simulink model "ROPOD_Control_Control_SIM"  (R2017b)
settings: Solver=VariableStepAuto  StartTime=0.0  StopTime=inf  RelTol=1e-3
values from neighbouring files (symbols this model uses):
  FFtheta_intia = 0    [init_model.m]
  FFxy_mass = 0*80    (= 0)    [init_model.m]
  flock_FFtheta_friction = 50    [init_model.m]
  flock_FFxy_friction = 100    [init_model.m]
  I_fhz_ddelta_cntr = 0    [init_model.m]
  I_fhz_dtheta_cntr = 0.3    [init_model.m]
  I_fhz_dtheta_flock_cntr = 0.1    [init_model.m]
  I_fhz_dvarphi_cntr = 0    [init_model.m]
  I_fhz_dxdy_cntr = 0.25    [init_model.m]
  I_fhz_dxdy_flock_cntr = 0.1    [init_model.m]
  K_gain_ddelta_cntr = 0.1    [init_model.m]
  K_gain_dtheta_cntr = 150    [init_model.m]
  K_gain_dtheta_flock_cntr = 100    [init_model.m]
  K_gain_dvarphi_cntr = 0.05    [init_model.m]
  K_gain_dxdy_cntr = 200    [init_model.m]
  K_gain_dxdy_flock_cntr = 200    [init_model.m]
  LL_wp_fhz_ddelta_cntr = 2    [init_model.m]
  LL_wp_fhz_dtheta_cntr = 20    [init_model.m]
  LL_wp_fhz_dtheta_flock_cntr = 20    [init_model.m]
  LL_wp_fhz_dvarphi_cntr = 10    [init_model.m]
  LL_wp_fhz_dxdy_cntr = 20    [init_model.m]
  LL_wp_fhz_dxdy_flock_cntr = 20    [init_model.m]
  LL_wz_fhz_ddelta_cntr = 2    [init_model.m]
  LL_wz_fhz_dtheta_cntr = 20    [init_model.m]
  LL_wz_fhz_dtheta_flock_cntr = 20    [init_model.m]
  LL_wz_fhz_dvarphi_cntr = 2    [init_model.m]
  LL_wz_fhz_dxdy_cntr = 20    [init_model.m]
  LL_wz_fhz_dxdy_flock_cntr = 20    [init_model.m]
  LPF_fhz_ddelta_cntr = 50    [init_model.m]
  LPF_fhz_ddelta_meas = 50    [init_model.m]
  LPF_fhz_dtheta_cntr = 100    [init_model.m]
  LPF_fhz_dtheta_flock_cntr = 40    [init_model.m]
  LPF_fhz_dvarphi_cntr = 50    [init_model.m]
  LPF_fhz_dvarphi_meas = 50    [init_model.m]
  LPF_fhz_dxdy_cntr = 100    [init_model.m]
  LPF_fhz_dxdy_flock_cntr = 40    [init_model.m]
  max_flock_acc_theta = 0.5    [init_model.m]
  max_flock_acc_xy = 0.5    [init_model.m]
  max_flock_vel_theta = 1.0    (= 1)    [init_model.m]
  max_flock_vel_xy = 1.0    (= 1)    [init_model.m]
  max_hw_tau = 7.0    (= 7)    [init_model.m]
  max_ropod_acc_theta = 1.6    [init_model.m]
  max_ropod_acc_xy = 2.0    (= 2)    [init_model.m]
  max_ropod_sw_force = 500    [init_model.m]
  max_ropod_sw_tau = 250    [init_model.m]
  max_ropod_vel_theta = 1.6    [init_model.m]
  max_ropod_vel_xy = 2.0    (= 2)    [init_model.m]
  max_sw_current = 10    [init_model.m]
  Nagents = 2    [init_model.m]
  Nwheels = 4    [Jqwl_numeric_function.m]    (also in S_matrix.m; extract_kinmodel_parameters.m; init_model.m; tau_optimal_dist_vec_fun.m)
  pivot_offs_sws = [0.0243    0.4689    0.3384    5.9050]    [init_model.m]
  ropod_kinmodel_pv = struct2array(ropod_kinmodel_param)    [set_ropod_KinModparams.m]
  ropod_position_inflock = [-1 0 3.1416]    [init_model.m]
  SW_COM1_ENABLE1 = hex2dec('0001')    [init_model.m]
  SW_COM1_ENABLE2 = hex2dec('0002')    [init_model.m]
  SW_COM1_MODE_TORQUE = bitshift(hex2dec('0000'),2)    [init_model.m]
  SW_COM1_MODE_VELOCITY = bitshift(hex2dec('0002'),2)    [init_model.m]
  SW_COM1_USE_TS = hex2dec('8000')    [init_model.m]
  Tinit = 2    [init_model.m]
  Ts = 0.001    [init_model.m]
  Tsflck = 0.01    [init_model.m]
undefined symbols (not defined in the file or in its folder): DiscIntNeverNeededParam, sw_tau_2_curr
libraries: simulink x80, cstblocks x30, dspsigops x12, dspnetwork x4
(part 2 of 6)

== system ROPOD_Control_Control_SIM/Flock_Control/Subscriber vel commands1 ==
  note: set 0 for testing
  note: if no vel commands are received after 0.5 sec, stop
  flock_kin_limits : Inport
  new_cmd : Inport  Port=2
  dq_flock_setp : Inport  Port=3
  Bus Selector1 : BusSelector  OutputSignals=max_acc_xy,max_vel_xy
  Bus Selector2 : BusSelector  OutputSignals=max_acc_xy,max_vel_xy
  Bus Selector3 : BusSelector  OutputSignals=max_acc_theta,max_vel_theta
  Compare To Constant : simulink/Logic and Bit Operations/Compare To Constant  relop=>=  const=0.5  OutDataTypeStr=boolean
  Constant : Constant  Value=0
  Constant1 : Constant  Value=0
  Constant2 : Constant  Value=0
  Demux : Demux  Outputs=3
  Digital Clock : DigitalClock  SampleTime=Tsflck
  Enabled Delay : Delay  DelayLength=1  ShowEnablePort=on  SampleTime=Tsflck
      settings: InputPortMap=u0,e6
  Gain{,1..5} (6 alike) : Gain  Gain=-1
  Gain6 : Gain
  Mux : Mux  Inputs=3
  Rate Limiter Dynamic : simulink/Discontinuities/Rate Limiter Dynamic
      settings: SourceProductName=Simulink
  Rate Limiter Dynamic1 : simulink/Discontinuities/Rate Limiter Dynamic
      settings: SourceProductName=Simulink
  Rate Limiter Dynamic2 : simulink/Discontinuities/Rate Limiter Dynamic
      settings: SourceProductName=Simulink
  Saturation Dynamic : simulink/Discontinuities/Saturation Dynamic  OutMin=[]  OutMax=[]  OutDataTypeStr=Inherit: Same as second input  OutDataType=fixdt(1, 16)  OutScaling=2^-10  DoSatur=off
  Saturation Dynamic1 : simulink/Discontinuities/Saturation Dynamic  OutMin=[]  OutMax=[]  OutDataTypeStr=Inherit: Same as second input  OutDataType=fixdt(1, 16)  OutScaling=2^-10  DoSatur=off
  Saturation Dynamic2 : simulink/Discontinuities/Saturation Dynamic  OutMin=[]  OutMax=[]  OutDataTypeStr=Inherit: Same as second input  OutDataType=fixdt(1, 16)  OutScaling=2^-10  DoSatur=off
  Subtract : Sum  Inputs=+-
  Switch : Switch  Criteria=u2 > Threshold
  Switch1 : Switch  Criteria=u2 > Threshold
  Switch2 : Switch  Criteria=u2 > Threshold
  dq_flock_setp_lim : Outport
  wires:
  Demux/1 -> Switch/3
  dq_flock_setp/1 -> Demux/1
  new_cmd/1 -> Enabled Delay/2
  Digital Clock/1 -> Enabled Delay/1, Subtract/1
  Enabled Delay/1 -> Subtract/2
  Subtract/1 -> Compare To Constant/1
  Constant/1 -> Switch/1
  Gain/1 -> Rate Limiter Dynamic/3
  Switch/1 -> Saturation Dynamic/2
  Gain1/1 -> Saturation Dynamic/3
  Saturation Dynamic/1 -> Rate Limiter Dynamic/2
  Switch1/1 -> Saturation Dynamic1/2
  Gain3/1 -> Saturation Dynamic1/3
  Constant1/1 -> Switch1/1
  Demux/2 -> Switch1/3
  Gain2/1 -> Rate Limiter Dynamic1/3
  Saturation Dynamic1/1 -> Rate Limiter Dynamic1/2
  Bus Selector2/1 -> Rate Limiter Dynamic1/1, Gain2/1  "<max_acc_xy>"
  Bus Selector2/2 -> Saturation Dynamic1/1, Gain3/1  "<max_vel_xy>"
  Bus Selector3/1 -> Rate Limiter Dynamic2/1, Gain4/1  "<max_acc_theta>"
  Saturation Dynamic2/1 -> Rate Limiter Dynamic2/2
  flock_kin_limits/1 -> Bus Selector3/1, Bus Selector2/1, Bus Selector1/1
  Switch2/1 -> Saturation Dynamic2/2
  Constant2/1 -> Switch2/1
  Demux/3 -> Switch2/3
  Gain5/1 -> Saturation Dynamic2/3
  Gain4/1 -> Rate Limiter Dynamic2/3
  Compare To Constant/1 -> Gain6/1
  Bus Selector3/2 -> Saturation Dynamic2/1, Gain5/1  "<max_vel_theta>"
  Mux/1 -> dq_flock_setp_lim/1
  Rate Limiter Dynamic/1 -> Mux/1
  Rate Limiter Dynamic1/1 -> Mux/2
  Rate Limiter Dynamic2/1 -> Mux/3
  Bus Selector1/2 -> Saturation Dynamic/1, Gain1/1  "<max_vel_xy>"
  Bus Selector1/1 -> Rate Limiter Dynamic/1, Gain/1  "<max_acc_xy>"
  Gain6/1 -> Switch2/2, Switch1/2, Switch/2

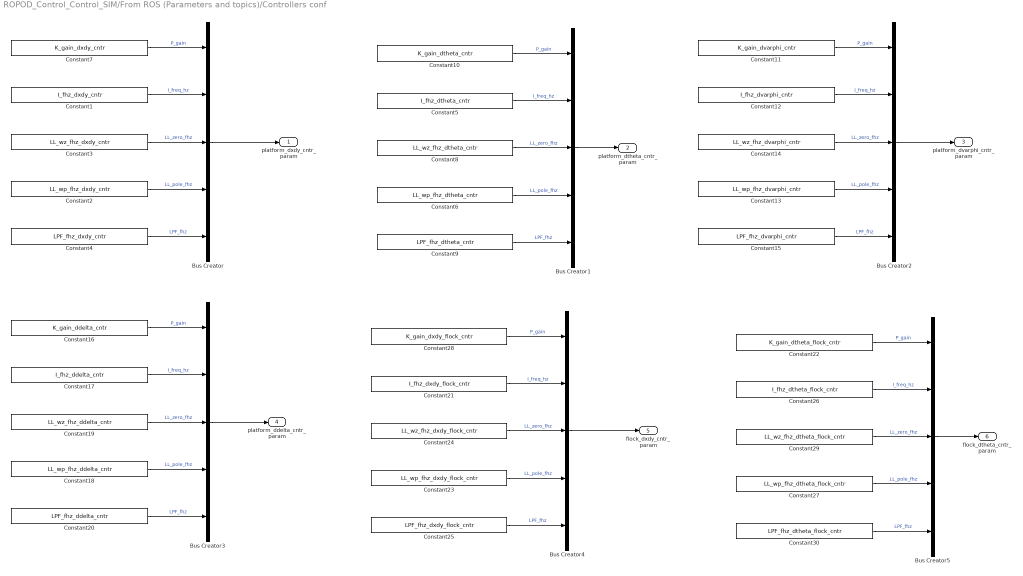
== system ROPOD_Control_Control_SIM/From ROS (Parameters and topics)/Controllers conf ==
  Bus Creator{,1..5} (6 alike) : BusCreator  Inputs=5
  Constant1 : Constant  Value=I_fhz_dxdy_cntr
  Constant10 : Constant  Value=K_gain_dtheta_cntr
  Constant11 : Constant  Value=K_gain_dvarphi_cntr
  Constant12 : Constant  Value=I_fhz_dvarphi_cntr
  Constant13 : Constant  Value=LL_wp_fhz_dvarphi_cntr
  Constant14 : Constant  Value=LL_wz_fhz_dvarphi_cntr
  Constant15 : Constant  Value=LPF_fhz_dvarphi_cntr
  Constant16 : Constant  Value=K_gain_ddelta_cntr
  Constant17 : Constant  Value=I_fhz_ddelta_cntr
  Constant18 : Constant  Value=LL_wp_fhz_ddelta_cntr
  Constant19 : Constant  Value=LL_wz_fhz_ddelta_cntr
  Constant2 : Constant  Value=LL_wp_fhz_dxdy_cntr
  Constant20 : Constant  Value=LPF_fhz_ddelta_cntr
  Constant21 : Constant  Value=I_fhz_dxdy_flock_cntr
  Constant22 : Constant  Value=K_gain_dtheta_flock_cntr
  Constant23 : Constant  Value=LL_wp_fhz_dxdy_flock_cntr
  Constant24 : Constant  Value=LL_wz_fhz_dxdy_flock_cntr
  Constant25 : Constant  Value=LPF_fhz_dxdy_flock_cntr
  Constant26 : Constant  Value=I_fhz_dtheta_flock_cntr
  Constant27 : Constant  Value=LL_wp_fhz_dtheta_flock_cntr
  Constant28 : Constant  Value=K_gain_dxdy_flock_cntr
  Constant29 : Constant  Value=LL_wz_fhz_dtheta_flock_cntr
  Constant3 : Constant  Value=LL_wz_fhz_dxdy_cntr
  Constant30 : Constant  Value=LPF_fhz_dtheta_flock_cntr
  Constant4 : Constant  Value=LPF_fhz_dxdy_cntr
  Constant5 : Constant  Value=I_fhz_dtheta_cntr
  Constant6 : Constant  Value=LL_wp_fhz_dtheta_cntr
  Constant7 : Constant  Value=K_gain_dxdy_cntr
  Constant8 : Constant  Value=LL_wz_fhz_dtheta_cntr
  Constant9 : Constant  Value=LPF_fhz_dtheta_cntr
  platform_dxdy_cntr_param : Outport
  platform_dtheta_cntr_param : Outport  Port=2
  platform_dvarphi_cntr_param : Outport  Port=3
  platform_ddelta_cntr_param : Outport  Port=4
  flock_dxdy_cntr_param : Outport  Port=5
  flock_dtheta_cntr_param : Outport  Port=6
  wires:
  Constant2/1 -> Bus Creator/4  "LL_pole_fhz"
  Constant4/1 -> Bus Creator/5  "LPF_fhz"
  Bus Creator/1 -> platform_dxdy_cntr_param/1
  Constant1/1 -> Bus Creator/2  "I_freq_hz"
  Constant3/1 -> Bus Creator/3  "LL_zero_fhz"
  Constant7/1 -> Bus Creator/1  "P_gain"
  Bus Creator1/1 -> platform_dtheta_cntr_param/1
  Bus Creator2/1 -> platform_dvarphi_cntr_param/1
  Constant5/1 -> Bus Creator1/2  "I_freq_hz"
  Constant6/1 -> Bus Creator1/4  "LL_pole_fhz"
  Constant10/1 -> Bus Creator1/1  "P_gain"
  Constant8/1 -> Bus Creator1/3  "LL_zero_fhz"
  Constant9/1 -> Bus Creator1/5  "LPF_fhz"
  Constant15/1 -> Bus Creator2/5  "LPF_fhz"
  Constant12/1 -> Bus Creator2/2  "I_freq_hz"
  Constant14/1 -> Bus Creator2/3  "LL_zero_fhz"
  Constant11/1 -> Bus Creator2/1  "P_gain"
  Constant13/1 -> Bus Creator2/4  "LL_pole_fhz"
  Constant17/1 -> Bus Creator3/2  "I_freq_hz"
  Constant20/1 -> Bus Creator3/5  "LPF_fhz"
  Constant18/1 -> Bus Creator3/4  "LL_pole_fhz"
  Constant19/1 -> Bus Creator3/3  "LL_zero_fhz"
  Bus Creator3/1 -> platform_ddelta_cntr_param/1
  Constant16/1 -> Bus Creator3/1  "P_gain"
  Constant30/1 -> Bus Creator5/5  "LPF_fhz"
  Constant27/1 -> Bus Creator5/4  "LL_pole_fhz"
  Bus Creator5/1 -> flock_dtheta_cntr_param/1
  Bus Creator4/1 -> flock_dxdy_cntr_param/1
  Constant28/1 -> Bus Creator4/1  "P_gain"
  Constant26/1 -> Bus Creator5/2  "I_freq_hz"
  Constant29/1 -> Bus Creator5/3  "LL_zero_fhz"
  Constant24/1 -> Bus Creator4/3  "LL_zero_fhz"
  Constant25/1 -> Bus Creator4/5  "LPF_fhz"
  Constant23/1 -> Bus Creator4/4  "LL_pole_fhz"
  Constant21/1 -> Bus Creator4/2  "I_freq_hz"
  Constant22/1 -> Bus Creator5/1  "P_gain"

== system ROPOD_Control_Control_SIM/From ROS (Parameters and topics)/ROS base conf ==
  Bus Creator : BusCreator  Inputs=4
  max_ropod_acc_theta : Constant  Value=max_ropod_acc_theta
  max_ropod_acc_xy : Constant  Value=max_ropod_acc_xy
  max_ropod_vel_theta : Constant  Value=max_ropod_vel_theta
  max_ropod_vel_xy : Constant  Value=max_ropod_vel_xy
  base_conf : Outport
  wires:
  max_ropod_acc_xy/1 -> Bus Creator/2  "max_acc_xy"
  max_ropod_vel_xy/1 -> Bus Creator/1  "max_vel_xy"
  Bus Creator/1 -> base_conf/1
  max_ropod_acc_theta/1 -> Bus Creator/4  "max_acc_theta"
  max_ropod_vel_theta/1 -> Bus Creator/3  "max_vel_theta"

== system ROPOD_Control_Control_SIM/From ROS (Parameters and topics)/flock kin limits ==
  Bus Creator : BusCreator  Inputs=4
  max_flock_acc_theta : Constant  Value=max_flock_acc_theta
  max_flock_acc_xy : Constant  Value=max_flock_acc_xy
  max_flock_vel_theta : Constant  Value=max_flock_vel_theta
  max_flock_vel_xy : Constant  Value=max_flock_vel_xy
  flock_kin_limits : Outport
  wires:
  max_flock_acc_xy/1 -> Bus Creator/2  "max_acc_xy"
  max_flock_vel_xy/1 -> Bus Creator/1  "max_vel_xy"
  Bus Creator/1 -> flock_kin_limits/1
  max_flock_acc_theta/1 -> Bus Creator/4  "max_acc_theta"
  max_flock_vel_theta/1 -> Bus Creator/3  "max_vel_theta"

== system ROPOD_Control_Control_SIM/RopodPlatformVelocityController/Platorm Velocity controller ==
  note: Mass Feedforward
  reset_int : Inport
  platform_dxdy_cntr_param : Inport  Port=2
  platform_dtheta_cntr_param : Inport  Port=3
  dqr_sp : Inport  Port=4
  dqr_loc : Inport  Port=5
  Demux : Demux  Outputs=3
  Demux1 : Demux  Outputs=3
  Discrete Derivative : simulink/Discrete/Discrete Derivative  gainval=1.0  ICPrevScaledInput=0.0  OutMin=[]  OutMax=[]  OutDataType=fixdt(1, 16)  OutScaling=2^-10  DoSatur=off
  G_I_LL_LPF Controller_X : Subsystem
  G_I_LL_LPF Controller_Y : Subsystem
  G_I_LL_LPF Controller_theta : Subsystem
  Gain : Gain  Gain=FFxy_mass
  Gain1 : Gain  Gain=FFxy_mass
  Gain2 : Gain  Gain=FFtheta_intia
  Mux : Mux  Inputs=3
  Mux1 : Mux  Inputs=3
  Sum : Sum  Inputs=|+-
  Sum1 : Sum  Inputs=++|
  w_platform_setp : Outport
  wires:
  Sum/1 -> Demux/1
  G_I_LL_LPF Controller_theta/1(Out) -> Mux/3
  Demux/1 -> G_I_LL_LPF Controller_X/2(In)
  Demux/2 -> G_I_LL_LPF Controller_Y/2(In)
  G_I_LL_LPF Controller_Y/1(Out) -> Mux/2
  G_I_LL_LPF Controller_X/1(Out) -> Mux/1
  Demux/3 -> G_I_LL_LPF Controller_theta/2(In)
  dqr_sp/1 -> Sum/1, Discrete Derivative/1
  dqr_loc/1 -> Sum/2
  [param_dxdy_cntr] -> G_I_LL_LPF Controller_X/1(param)
  [param_dxdy_cntr] -> G_I_LL_LPF Controller_Y/1(param)
  [param_dtheta_cntr] -> G_I_LL_LPF Controller_theta/1(param)
  reset_int/1 -> [reset_int_cntr]
  [reset_int_cntr] -> G_I_LL_LPF Controller_X/3(reset_integrator)
  [reset_int_cntr] -> G_I_LL_LPF Controller_Y/3(reset_integrator)
  platform_dxdy_cntr_param/1 -> [param_dxdy_cntr]
  platform_dtheta_cntr_param/1 -> [param_dtheta_cntr]
  [reset_int_cntr] -> G_I_LL_LPF Controller_theta/3(reset_integrator)
  Discrete Derivative/1 -> Demux1/1
  Demux1/1 -> Gain/1
  Gain/1 -> Mux1/1
  Demux1/2 -> Gain1/1
  Gain1/1 -> Mux1/2
  Demux1/3 -> Gain2/1
  Gain2/1 -> Mux1/3
  Sum1/1 -> w_platform_setp/1
  Mux1/1 -> Sum1/1
  Mux/1 -> Sum1/2

== system ROPOD_Control_Control_SIM/RopodPlatformVelocityController/Subscriber vel commands1 ==
  note: set 0 for testing
  note: if no vel commands are received after 0.5 sec, stop
  base_conf : Inport
  new_cmd : Inport  Port=2
  dq_setp : Inport  Port=3
  Bus Selector1 : BusSelector  OutputSignals=max_acc_xy,max_vel_xy
  Bus Selector2 : BusSelector  OutputSignals=max_acc_xy,max_vel_xy
  Bus Selector3 : BusSelector  OutputSignals=max_acc_theta,max_vel_theta
  Compare To Constant : simulink/Logic and Bit Operations/Compare To Constant  relop=>=  const=0.5  OutDataTypeStr=boolean
  Constant : Constant  Value=0  SampleTime=Ts
  Constant1 : Constant  Value=0
  Constant2 : Constant  Value=0
  Demux : Demux  Outputs=3
  Digital Clock : DigitalClock  SampleTime=Ts
  Enabled Delay : Delay  DelayLength=1  ShowEnablePort=on  SampleTime=Ts
      settings: InputPortMap=u0,e6
  Gain{,1..5} (6 alike) : Gain  Gain=-1
  Gain6 : Gain
  Mux : Mux  Inputs=3
  Rate Limiter Dynamic : simulink/Discontinuities/Rate Limiter Dynamic
      settings: SourceProductName=Simulink
  Rate Limiter Dynamic1 : simulink/Discontinuities/Rate Limiter Dynamic
      settings: SourceProductName=Simulink
  Rate Limiter Dynamic2 : simulink/Discontinuities/Rate Limiter Dynamic
      settings: SourceProductName=Simulink
  Saturation Dynamic : simulink/Discontinuities/Saturation Dynamic  OutMin=[]  OutMax=[]  OutDataTypeStr=Inherit: Same as second input  OutDataType=fixdt(1, 16)  OutScaling=2^-10  DoSatur=off
  Saturation Dynamic1 : simulink/Discontinuities/Saturation Dynamic  OutMin=[]  OutMax=[]  OutDataTypeStr=Inherit: Same as second input  OutDataType=fixdt(1, 16)  OutScaling=2^-10  DoSatur=off
  Saturation Dynamic2 : simulink/Discontinuities/Saturation Dynamic  OutMin=[]  OutMax=[]  OutDataTypeStr=Inherit: Same as second input  OutDataType=fixdt(1, 16)  OutScaling=2^-10  DoSatur=off
  Subtract : Sum  Inputs=+-
  Switch : Switch  Criteria=u2 > Threshold
  Switch1 : Switch  Criteria=u2 > Threshold
  Switch2 : Switch  Criteria=u2 > Threshold
  dq_loc_sp : Outport
  wires:
  Demux/1 -> Switch/3
  dq_setp/1 -> Demux/1
  new_cmd/1 -> Enabled Delay/2
  Digital Clock/1 -> Enabled Delay/1, Subtract/1
  Enabled Delay/1 -> Subtract/2
  Subtract/1 -> Compare To Constant/1
  Constant/1 -> Switch/1
  Gain/1 -> Rate Limiter Dynamic/3
  Switch/1 -> Saturation Dynamic/2
  Gain1/1 -> Saturation Dynamic/3
  Saturation Dynamic/1 -> Rate Limiter Dynamic/2
  Switch1/1 -> Saturation Dynamic1/2
  Gain3/1 -> Saturation Dynamic1/3
  Constant1/1 -> Switch1/1
  Demux/2 -> Switch1/3
  Gain2/1 -> Rate Limiter Dynamic1/3
  Saturation Dynamic1/1 -> Rate Limiter Dynamic1/2
  Bus Selector2/1 -> Rate Limiter Dynamic1/1, Gain2/1  "<max_acc_xy>"
  Bus Selector2/2 -> Saturation Dynamic1/1, Gain3/1  "<max_vel_xy>"
  Bus Selector3/1 -> Rate Limiter Dynamic2/1, Gain4/1  "<max_acc_theta>"
  Saturation Dynamic2/1 -> Rate Limiter Dynamic2/2
  base_conf/1 -> Bus Selector3/1, Bus Selector2/1, Bus Selector1/1
  Switch2/1 -> Saturation Dynamic2/2
  Constant2/1 -> Switch2/1
  Demux/3 -> Switch2/3
  Gain5/1 -> Saturation Dynamic2/3
  Gain4/1 -> Rate Limiter Dynamic2/3
  Compare To Constant/1 -> Gain6/1
  Bus Selector3/2 -> Saturation Dynamic2/1, Gain5/1  "<max_vel_theta>"
  Mux/1 -> dq_loc_sp/1
  Rate Limiter Dynamic/1 -> Mux/1
  Rate Limiter Dynamic1/1 -> Mux/2
  Rate Limiter Dynamic2/1 -> Mux/3
  Bus Selector1/2 -> Saturation Dynamic/1, Gain1/1  "<max_vel_xy>"
  Bus Selector1/1 -> Rate Limiter Dynamic/1, Gain/1  "<max_acc_xy>"
  Gain6/1 -> Switch2/2, Switch1/2, Switch/2

== system ROPOD_Control_Control_SIM/RopodProcessWheelSensorData/Odometry and Measurement model 4SW ==
  note: This output is only useful when using ros
      | This data is fed to /odom/pose
  note: This part is in global coordinates
  note: This part is in local coordinates
  param_in : Inport
  ena_w : Inport  Port=2
  dvarphi : Inport  Port=3
  delta : Inport  Port=4
  Discrete-Time Integrator : DiscreteIntegrator  InitialConditionSetting=State (most efficient)  SampleTime=Ts  ICPrevOutput=DiscIntNeverNeededParam  ICPrevScaledInput=DiscIntNeverNeededParam
  Jqwl_numeric : MATLAB Function  TreatAsAtomicUnit=on
  Selector3 : Selector  InputPortWidth=3  IndexOptions=Index vector (dialog)  Indices=3  OutputSizes=1
  Signal Specification : SignalSpecification  Dimensions=[3 1]
  pos_rot_matrix : MATLAB Function  TreatAsAtomicUnit=on
  odom_robot_pose : Outport
  odom_robot_twist : Outport  Port=2
  wires:
  Jqwl_numeric/1(v) -> Signal Specification/1
  param_in/1 -> Jqwl_numeric/1(ropod_kinmodel_param_vec)
  delta/1 -> Jqwl_numeric/2(delta)
  Signal Specification/1 -> pos_rot_matrix/1(dqr_loc), odom_robot_twist/1
  Selector3/1 -> pos_rot_matrix/2(theta_odom)
  pos_rot_matrix/1(dqr_glb) -> Discrete-Time Integrator/1
  Discrete-Time Integrator/1 -> odom_robot_pose/1, Selector3/1
  dvarphi/1 -> Jqwl_numeric/3(dvarphi)
  ena_w/1 -> Jqwl_numeric/4(ena_w)

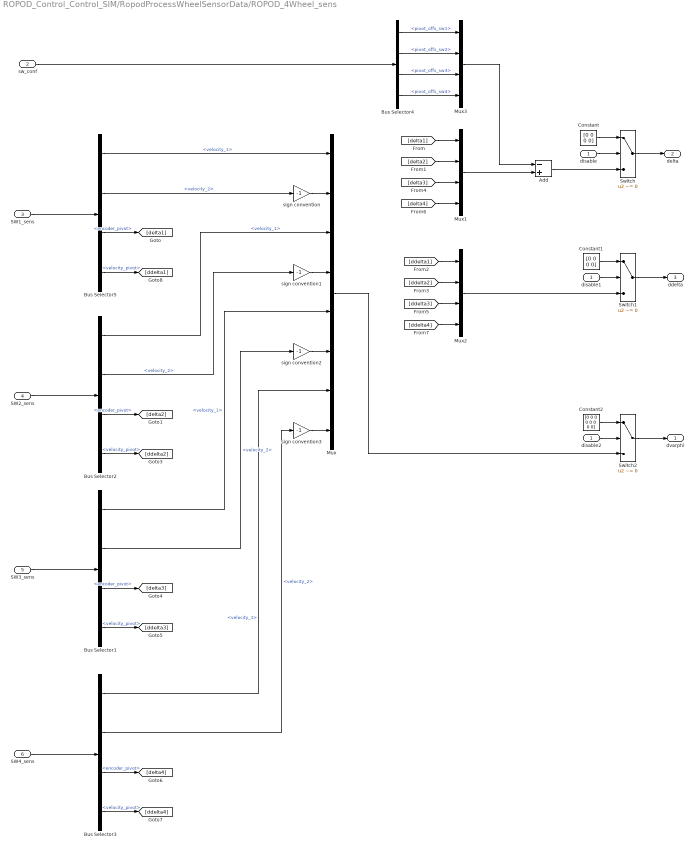
== system ROPOD_Control_Control_SIM/RopodProcessWheelSensorData/ROPOD_4Wheel_sens ==
  disable : Inport
  sw_conf : Inport  Port=2
  SW1_sens : Inport  Port=3
  SW2_sens : Inport  Port=4
  SW3_sens : Inport  Port=5
  SW4_sens : Inport  Port=6
  Add : Sum  Inputs=-+
  Bus Selector{1..3,5} (4 alike) : BusSelector  OutputSignals=velocity_1,velocity_2,encoder_pivot,velocity_pivot
  Bus Selector4 : BusSelector  OutputSignals=pivot_offs_sw1,pivot_offs_sw2,pivot_offs_sw3,pivot_offs_sw4
  Constant : Constant  Value=[0 0 0 0]
  Constant1 : Constant  Value=[0 0 0 0]
  Constant2 : Constant  Value=[0 0 0 0 0 0 0 0]
  Mux : Mux  Inputs=8
  Mux1 : Mux
  Mux2 : Mux
  Mux3 : Mux
  Switch : Switch  Criteria=u2 ~= 0
  Switch1 : Switch  Criteria=u2 ~= 0
  Switch2 : Switch  Criteria=u2 ~= 0
  disable1 : InportShadow
  disable2 : InportShadow
  sign convention{,1..3} (4 alike) : Gain  Gain=-1
  dvarphi : Outport
  delta : Outport  Port=2
  ddelta : Outport  Port=3
  wires:
  SW1_sens/1 -> Bus Selector5/1
  SW2_sens/1 -> Bus Selector2/1
  Bus Selector5/1 -> Mux/1  "<velocity_1>"
  Bus Selector5/2 -> sign convention/1  "<velocity_2>"
  Bus Selector2/1 -> Mux/3  "<velocity_1>"
  Bus Selector2/2 -> sign convention1/1  "<velocity_2>"
  Bus Selector2/3 -> [delta2]  "<encoder_pivot>"
  [delta1] -> Mux1/1
  [delta2] -> Mux1/2
  Bus Selector2/4 -> [ddelta2]  "<velocity_pivot>"
  [ddelta2] -> Mux2/2
  [ddelta1] -> Mux2/1
  Bus Selector1/4 -> [ddelta3]  "<velocity_pivot>"
  Bus Selector1/3 -> [delta3]  "<encoder_pivot>"
  Bus Selector1/2 -> sign convention2/1  "<velocity_2>"
  Bus Selector1/1 -> Mux/5  "<velocity_1>"
  SW3_sens/1 -> Bus Selector1/1
  [delta3] -> Mux1/3
  [ddelta3] -> Mux2/3
  SW4_sens/1 -> Bus Selector3/1
  Bus Selector3/1 -> Mux/7  "<velocity_1>"
  Bus Selector3/2 -> sign convention3/1  "<velocity_2>"
  Bus Selector3/3 -> [delta4]  "<encoder_pivot>"
  Bus Selector3/4 -> [ddelta4]  "<velocity_pivot>"
  [delta4] -> Mux1/4
  [ddelta4] -> Mux2/4
  Mux1/1 -> Add/2
  Mux3/1 -> Add/1
  sw_conf/1 -> Bus Selector4/1
  Bus Selector4/1 -> Mux3/1  "<pivot_offs_sw1>"
  Bus Selector4/2 -> Mux3/2  "<pivot_offs_sw2>"
  Bus Selector4/3 -> Mux3/3  "<pivot_offs_sw3>"
  Bus Selector4/4 -> Mux3/4  "<pivot_offs_sw4>"
  Bus Selector5/3 -> [delta1]  "<encoder_pivot>"
  Bus Selector5/4 -> [ddelta1]  "<velocity_pivot>"
  sign convention/1 -> Mux/2
  sign convention1/1 -> Mux/4
  sign convention2/1 -> Mux/6
  sign convention3/1 -> Mux/8
  Add/1 -> Switch/3
  Switch/1 -> delta/1
  disable/1 -> Switch/2
  Constant/1 -> Switch/1
  Switch1/1 -> ddelta/1
  Mux2/1 -> Switch1/3
  Constant1/1 -> Switch1/1
  disable1/1 -> Switch1/2
  disable2/1 -> Switch2/2
  Constant2/1 -> Switch2/1
  Mux/1 -> Switch2/3
  Switch2/1 -> dvarphi/1

== system ROPOD_Control_Control_SIM/RopodTorqueDistribution/Inverse Kinematics 4SW ==
  param_in : Inport
  dqr_sp : Inport  Port=2
  delta : Inport  Port=3
  Gl_matrix : MATLAB Function  TreatAsAtomicUnit=on
  Product3 : Product  Multiplication=Matrix(*)
  Selector2 : Selector  IndexMode=Zero-based  InputPortWidth=3+3*Nwheels  IndexOptions=Index vector (dialog)  Indices=[3+Nwheels:3+3*Nwheels-1]  OutputSizes=1
  wheel_vel_sp : Outport
  wires:
  param_in/1 -> Gl_matrix/1(ropod_kinmodel_param_vec)
  Gl_matrix/1(Gl) -> Product3/1
  Product3/1 -> Selector2/1
  delta/1 -> Gl_matrix/2(delta)
  dqr_sp/1 -> Product3/2
  Selector2/1 -> wheel_vel_sp/1

== system ROPOD_Control_Control_SIM/RopodTorqueDistribution/ROPOD 4SW ==
  note: disable = 0, current = 1, initialize = 2
  sw_conf : Inport
  ropod_cntr_mode : Inport  Port=2
  varphi_tau_setp : Inport  Port=3
  Bus Creator : BusCreator  Commented=on  Inputs=4
  Bus Creator1 : BusCreator  Commented=on  Inputs=4
  Gain3 : Gain  Gain=sw_tau_2_curr
  Initialization switch : Subsystem
  ROPOD_4Wheel_sens_own_vel_filter : Subsystem  Commented=on
  ROPOD_4Wheel_torque_cmd : Subsystem
  To File : ToFile  Commented=on  Filename=all_wheel_out_data  MatrixName=all_wheel_out_data
  To File2 : ToFile  Commented=on  Filename=all_wheel_in_data  MatrixName=all_wheel_in_data
  empywheel : Subsystem  Commented=on
  SW1_cmd : Outport
  SW2_cmd : Outport  Port=2
  SW3_cmd : Outport  Port=3
  SW4_cmd : Outport  Port=4
  wires:
  ROPOD_4Wheel_torque_cmd/4(SW4_cmd) -> SW4_cmd/1, Bus Creator1/4  "SW4_cmd"
  ROPOD_4Wheel_torque_cmd/1(SW1_cmd) -> SW1_cmd/1, Bus Creator1/1  "SW1_cmd"
  ROPOD_4Wheel_torque_cmd/3(SW3_cmd) -> SW3_cmd/1, Bus Creator1/3  "SW3_cmd"
  sw_conf/1 -> ROPOD_4Wheel_torque_cmd/1(sw_conf)
  ROPOD_4Wheel_torque_cmd/2(SW2_cmd) -> SW2_cmd/1, Bus Creator1/2  "SW2_cmd"
  Bus Creator/1 -> To File/1
  Bus Creator1/1 -> To File2/1
  varphi_tau_setp/1 -> Gain3/1
  Gain3/1 -> Initialization switch/2(curr_setp)
  ropod_cntr_mode/1 -> Initialization switch/1(ropod_cntr_mode)
  Initialization switch/1(SW_cntr_mode) -> ROPOD_4Wheel_torque_cmd/2(cntr_mode)
  Initialization switch/2(wheel_setp) -> ROPOD_4Wheel_torque_cmd/3(wheel_setp)

== system ROPOD_Control_Control_SIM/RopodTorqueDistribution/Torque distribution ==
  w_platform_setp : Inport
  ropod_kinmodel_pv : Inport  Port=2
  sw_conf : Inport  Port=3
  delta : Inport  Port=4
  ena_w : Inport  Port=5
  Add : Sum  Inputs=+-
  Bus Selector1 : BusSelector  OutputSignals=max_current
  Gain3 : Gain  Gain=1/sw_tau_2_curr
  Gl_matrices : MATLAB Function  TreatAsAtomicUnit=on
  Product1 : Product  Multiplication=Matrix(*)
  Signal Specification : SignalSpecification  Dimensions=[3 1]
  Terminator : Terminator
  Terminator1 : Terminator
  Terminator2 : Terminator
  To File1 : ToFile  Commented=on  Filename=dist_check_tau_setp.mat  MatrixName=dist_check_tau_setp
  platform_forces_2_tau_dist_optimal : MATLAB Function  TreatAsAtomicUnit=on
  varphi_tau_setp_out : Outport
  wires:
  Gl_matrices/3(GtSl) -> [GtSl_matrix]
  Gl_matrices/1(Gl) -> Terminator/1
  delta/1 -> Gl_matrices/2(delta)
  Gl_matrices/2(Gtl) -> Terminator1/1
  ropod_kinmodel_pv/1 -> Gl_matrices/1(ropod_kinmodel_param_vec)
  Bus Selector1/1 -> Gain3/1  "<max_current>"
  sw_conf/1 -> Bus Selector1/1
  Gain3/1 -> platform_forces_2_tau_dist_optimal/4(tau_max)
  ena_w/1 -> platform_forces_2_tau_dist_optimal/3(ena_w)
  [GtSl_matrix] -> platform_forces_2_tau_dist_optimal/1(GtSl), Product1/1
  w_platform_setp/1 -> Signal Specification/1
  platform_forces_2_tau_dist_optimal/2(taubody_sc) -> Terminator2/1
  platform_forces_2_tau_dist_optimal/1(Ttaud) -> Product1/2, varphi_tau_setp_out/1
  Product1/1 -> Add/1
  Add/1 -> To File1/1
  Signal Specification/1 -> platform_forces_2_tau_dist_optimal/2(taubody), Add/2

== system ROPOD_Control_Control_SIM/RopodTorqueDistribution/pivot damping cntr ==
  platform_ddelta_cntr_param : Inport
  disable : Inport  Port=2
  ddelta_ref : Inport  Port=3
  ddelta : Inport  Port=4
  ena_w : Inport  Port=5
  Pivot controller : Subsystem
  Sum : Sum  Inputs=|+-
  varphi_tau_setp_out : Outport
  wires:
  Pivot controller/1(varphi_tau_setp) -> varphi_tau_setp_out/1
  ena_w/1 -> Pivot controller/2(ena_w)
  Sum/1 -> Pivot controller/1(dvarphi_error)
  ddelta/1 -> Sum/2
  disable/1 -> Pivot controller/4(reset_int)
  platform_ddelta_cntr_param/1 -> Pivot controller/3(platform_dvarphi_cntr_param)
  ddelta_ref/1 -> Sum/1

== system ROPOD_Control_Control_SIM/RopodTorqueDistribution/wheel flip compensation ==
  varphi_tau_sp_in : Inport
  ropod_kin_param : Inport  Port=2
  flip_comp_factor : Inport  Port=3
  sw_conf : Inport  Port=4
  Bus Selector : BusSelector  OutputSignals=max_current
  Constant : Constant  Value=10
  Demux : Demux  Outputs=8
  Gain3 : Gain  Gain=1/sw_tau_2_curr
  MATLAB Function1 : MATLAB Function  TreatAsAtomicUnit=on
  MATLAB Function2 : MATLAB Function  TreatAsAtomicUnit=on
  MATLAB Function3 : MATLAB Function  TreatAsAtomicUnit=on
  MATLAB Function4 : MATLAB Function  TreatAsAtomicUnit=on
  Mux : Mux  Inputs=8
  Terminator{,1..3} (4 alike) : Terminator
  varphi_tau_sp_out : Outport
  wires:
  varphi_tau_sp_in/1 -> Demux/1
  ropod_kin_param/1 -> [ropod_kin_param]
  flip_comp_factor/1 -> [kmax]
  Demux/2 -> MATLAB Function4/2(tr)
  Demux/1 -> MATLAB Function4/1(tl)
  [kmax] -> MATLAB Function4/4(kmax)
  [ropod_kin_param] -> MATLAB Function4/3(ropod_kinmodel_param_vec)
  MATLAB Function4/1(tl_out) -> Mux/1
  MATLAB Function4/2(tr_out) -> Mux/2
  MATLAB Function4/3(sc) -> Terminator/1
  Mux/1 -> varphi_tau_sp_out/1
  Constant/1 -> [Fthr]
  [Fthr] -> MATLAB Function4/5(Fthr)
  sw_conf/1 -> Bus Selector/1
  Bus Selector/1 -> Gain3/1  "<max_current>"
  Gain3/1 -> [tau_max]
  [tau_max] -> MATLAB Function4/6(tau_max)
  MATLAB Function1/3(sc) -> Terminator1/1
  Demux/4 -> MATLAB Function1/2(tr)
  [Fthr] -> MATLAB Function1/5(Fthr)
  MATLAB Function1/2(tr_out) -> Mux/4
  Demux/3 -> MATLAB Function1/1(tl)
  [ropod_kin_param] -> MATLAB Function1/3(ropod_kinmodel_param_vec)
  [kmax] -> MATLAB Function1/4(kmax)
  MATLAB Function1/1(tl_out) -> Mux/3
  [tau_max] -> MATLAB Function1/6(tau_max)
  Demux/7 -> MATLAB Function3/1(tl)
  [kmax] -> MATLAB Function3/4(kmax)
  Demux/8 -> MATLAB Function3/2(tr)
  [ropod_kin_param] -> MATLAB Function2/3(ropod_kinmodel_param_vec)
  MATLAB Function3/2(tr_out) -> Mux/8
  Demux/5 -> MATLAB Function2/1(tl)
  [tau_max] -> MATLAB Function2/6(tau_max)
  [tau_max] -> MATLAB Function3/6(tau_max)
  [Fthr] -> MATLAB Function2/5(Fthr)
  MATLAB Function3/1(tl_out) -> Mux/7
  [Fthr] -> MATLAB Function3/5(Fthr)
  MATLAB Function2/3(sc) -> Terminator2/1
  MATLAB Function3/3(sc) -> Terminator3/1
  MATLAB Function2/2(tr_out) -> Mux/6
  [kmax] -> MATLAB Function2/4(kmax)
  Demux/6 -> MATLAB Function2/2(tr)
  [ropod_kin_param] -> MATLAB Function3/3(ropod_kinmodel_param_vec)
  MATLAB Function2/1(tl_out) -> Mux/5

== system ROPOD_Control_Control_SIM/RopodTorqueDistribution/wheel vel cntr ==
  platform_dxdy_cntr_param : Inport
  disable : Inport  Port=2
  dvarphi_sp : Inport  Port=3
  ena_w : Inport  Port=4
  dvarphi : Inport  Port=5
  Sum : Sum  Inputs=-+|
  Wheels Velocity controller : Subsystem
  varphi_tau_setp_out : Outport
  wires:
  Wheels Velocity controller/1(varphi_tau_setp) -> varphi_tau_setp_out/1
  ena_w/1 -> Wheels Velocity controller/2(ena_w)
  Sum/1 -> Wheels Velocity controller/1(dvarphi_error)
  dvarphi/1 -> Sum/1
  dvarphi_sp/1 -> Sum/2
  disable/1 -> Wheels Velocity controller/4(reset_int)
  platform_dxdy_cntr_param/1 -> Wheels Velocity controller/3(platform_dvarphi_cntr_param)

== system ROPOD_Control_Control_SIM/Subsystem/Ropod kinematic parameters ==
  ropod_kinmodel_pv : Constant  Value=ropod_kinmodel_pv
  ropod_kin_param : Outport
  wires:
  ropod_kinmodel_pv/1 -> ropod_kin_param/1

== system ROPOD_Control_Control_SIM/Subsystem/Smart wheels conf1 ==
  Bus Creator : BusCreator  Inputs=8
  LPF_fhz_ddelta_meas : Constant  Value=LPF_fhz_ddelta_meas
  LPF_fhz_dvarphi_meas : Constant  Value=LPF_fhz_dvarphi_meas
  enable : Constant
  max_current : Constant  Value=max_sw_current
  pivot_offset_sw1 : Constant  Value=pivot_offs_sws(1)
  pivot_offset_sw2 : Constant  Value=pivot_offs_sws(2)
  pivot_offset_sw3 : Constant  Value=pivot_offs_sws(3)
  pivot_offset_sw4 : Constant  Value=pivot_offs_sws(4)
  sw_conf : Outport
  wires:
  enable/1 -> Bus Creator/1  "enable"
  Bus Creator/1 -> sw_conf/1
  max_current/1 -> Bus Creator/2  "max_current"
  pivot_offset_sw1/1 -> Bus Creator/3  "pivot_offs_sw1"
  pivot_offset_sw2/1 -> Bus Creator/4  "pivot_offs_sw2"
  pivot_offset_sw3/1 -> Bus Creator/5  "pivot_offs_sw3"
  pivot_offset_sw4/1 -> Bus Creator/6  "pivot_offs_sw4"
  LPF_fhz_dvarphi_meas/1 -> Bus Creator/7  "dvarphi_LPF_fhz"
  LPF_fhz_ddelta_meas/1 -> Bus Creator/8  "ddelta_LPF_fhz"

== system ROPOD_Control_Control_SIM/Flock_Control/Flock Velocity controller/G_I_LL_LPF Controller_flock_Theta ==
  param : Inport
  In : Inport  Port=2
  reset_integrator : Inport  Port=3
  Bus Selector : BusSelector  OutputSignals=P_gain,I_freq_hz,LL_zero_fhz,LL_pole_fhz,LPF_fhz
  Discrete Varying Lowpass3 : cstblocks/Linear Parameter Varying/Discrete Varying Lowpass  N=1  w0=0  Ts=Tsflck
      settings: SourceProductName=Control System Toolbox  SourceProductBaseCode=CT
  Gain2 : Gain  Gain=2*pi
  Product5 : Product
  Shapeit Integrator (Tustin) : Subsystem
  Shapeit Lead-Lag (Tustin) : Subsystem
  Out : Outport
  wires:
  Gain2/1 -> Discrete Varying Lowpass3/2
  Product5/1 -> Shapeit Integrator (Tustin)/1(In)
  Discrete Varying Lowpass3/1 -> Out/1
  Shapeit Integrator (Tustin)/1(Out) -> Shapeit Lead-Lag (Tustin)/1(In)
  Bus Selector/1 -> Product5/2  "<P_gain>"
  Bus Selector/2 -> Shapeit Integrator (Tustin)/2(I_fhz)  "<I_freq_hz>"
  param/1 -> Bus Selector/1
  Bus Selector/5 -> Gain2/1  "<LPF_fhz>"
  Bus Selector/4 -> Shapeit Lead-Lag (Tustin)/3(fp)  "<LL_pole_fhz>"
  reset_integrator/1 -> Shapeit Integrator (Tustin)/3(reset)
  Bus Selector/3 -> Shapeit Lead-Lag (Tustin)/2(fz)  "<LL_zero_fhz>"
  Shapeit Lead-Lag (Tustin)/1(Out) -> Discrete Varying Lowpass3/1
  In/1 -> Product5/1

== system ROPOD_Control_Control_SIM/Flock_Control/Flock Velocity controller/G_I_LL_LPF Controller_flock_X ==
  param : Inport
  In : Inport  Port=2
  reset_integrator : Inport  Port=3
  Bus Selector : BusSelector  OutputSignals=P_gain,I_freq_hz,LL_zero_fhz,LL_pole_fhz,LPF_fhz
  Discrete Varying Lowpass3 : cstblocks/Linear Parameter Varying/Discrete Varying Lowpass  N=1  w0=0  Ts=Tsflck
      settings: SourceProductName=Control System Toolbox  SourceProductBaseCode=CT
  Gain2 : Gain  Gain=2*pi
  Product5 : Product
  Shapeit Integrator (Tustin) : Subsystem
  Shapeit Lead-Lag (Tustin) : Subsystem
  Out : Outport
  wires:
  Gain2/1 -> Discrete Varying Lowpass3/2
  Product5/1 -> Shapeit Integrator (Tustin)/1(In)
  Discrete Varying Lowpass3/1 -> Out/1
  Shapeit Integrator (Tustin)/1(Out) -> Shapeit Lead-Lag (Tustin)/1(In)
  Bus Selector/1 -> Product5/2  "<P_gain>"
  Bus Selector/2 -> Shapeit Integrator (Tustin)/2(I_fhz)  "<I_freq_hz>"
  param/1 -> Bus Selector/1
  Bus Selector/5 -> Gain2/1  "<LPF_fhz>"
  Bus Selector/4 -> Shapeit Lead-Lag (Tustin)/3(fp)  "<LL_pole_fhz>"
  reset_integrator/1 -> Shapeit Integrator (Tustin)/3(reset)
  Bus Selector/3 -> Shapeit Lead-Lag (Tustin)/2(fz)  "<LL_zero_fhz>"
  Shapeit Lead-Lag (Tustin)/1(Out) -> Discrete Varying Lowpass3/1
  In/1 -> Product5/1

== system ROPOD_Control_Control_SIM/Flock_Control/Flock Velocity controller/G_I_LL_LPF Controller_flock_Y ==
  param : Inport
  In : Inport  Port=2
  reset_integrator : Inport  Port=3
  Bus Selector : BusSelector  OutputSignals=P_gain,I_freq_hz,LL_zero_fhz,LL_pole_fhz,LPF_fhz
  Discrete Varying Lowpass3 : cstblocks/Linear Parameter Varying/Discrete Varying Lowpass  N=1  w0=0  Ts=Tsflck
      settings: SourceProductName=Control System Toolbox  SourceProductBaseCode=CT
  Gain2 : Gain  Gain=2*pi
  Product5 : Product
  Shapeit Integrator (Tustin) : Subsystem
  Shapeit Lead-Lag (Tustin) : Subsystem
  Out : Outport
  wires:
  Gain2/1 -> Discrete Varying Lowpass3/2
  Product5/1 -> Shapeit Integrator (Tustin)/1(In)
  Discrete Varying Lowpass3/1 -> Out/1
  Shapeit Integrator (Tustin)/1(Out) -> Shapeit Lead-Lag (Tustin)/1(In)
  Bus Selector/1 -> Product5/2  "<P_gain>"
  Bus Selector/2 -> Shapeit Integrator (Tustin)/2(I_fhz)  "<I_freq_hz>"
  param/1 -> Bus Selector/1
  Bus Selector/5 -> Gain2/1  "<LPF_fhz>"
  Bus Selector/4 -> Shapeit Lead-Lag (Tustin)/3(fp)  "<LL_pole_fhz>"
  reset_integrator/1 -> Shapeit Integrator (Tustin)/3(reset)
  Bus Selector/3 -> Shapeit Lead-Lag (Tustin)/2(fz)  "<LL_zero_fhz>"
  Shapeit Lead-Lag (Tustin)/1(Out) -> Discrete Varying Lowpass3/1
  In/1 -> Product5/1

== system ROPOD_Control_Control_SIM/RopodPlatformVelocityController/Platorm Velocity controller/G_I_LL_LPF Controller_X ==
  param : Inport
  In : Inport  Port=2
  reset_integrator : Inport  Port=3
  Bus Selector : BusSelector  OutputSignals=P_gain,I_freq_hz,LL_zero_fhz,LL_pole_fhz,LPF_fhz
  Discrete Varying Lowpass3 : cstblocks/Linear Parameter Varying/Discrete Varying Lowpass  N=1  w0=0  Ts=Ts
      settings: SourceProductName=Control System Toolbox  SourceProductBaseCode=CT
  Gain2 : Gain  Gain=2*pi
  Product5 : Product
  Shapeit Integrator (Tustin) : Subsystem
  Shapeit Lead-Lag (Tustin) : Subsystem
  Out : Outport
  wires:
  Gain2/1 -> Discrete Varying Lowpass3/2
  Product5/1 -> Shapeit Integrator (Tustin)/1(In)
  Discrete Varying Lowpass3/1 -> Out/1
  Shapeit Integrator (Tustin)/1(Out) -> Shapeit Lead-Lag (Tustin)/1(In)
  Bus Selector/1 -> Product5/2  "<P_gain>"
  Bus Selector/2 -> Shapeit Integrator (Tustin)/2(I_fhz)  "<I_freq_hz>"
  param/1 -> Bus Selector/1
  Bus Selector/5 -> Gain2/1  "<LPF_fhz>"
  Bus Selector/4 -> Shapeit Lead-Lag (Tustin)/3(fp)  "<LL_pole_fhz>"
  reset_integrator/1 -> Shapeit Integrator (Tustin)/3(reset)
  Bus Selector/3 -> Shapeit Lead-Lag (Tustin)/2(fz)  "<LL_zero_fhz>"
  Shapeit Lead-Lag (Tustin)/1(Out) -> Discrete Varying Lowpass3/1
  In/1 -> Product5/1

== system ROPOD_Control_Control_SIM/RopodPlatformVelocityController/Platorm Velocity controller/G_I_LL_LPF Controller_Y ==
  param : Inport
  In : Inport  Port=2
  reset_integrator : Inport  Port=3
  Bus Selector : BusSelector  OutputSignals=P_gain,I_freq_hz,LL_zero_fhz,LL_pole_fhz,LPF_fhz
  Discrete Varying Lowpass3 : cstblocks/Linear Parameter Varying/Discrete Varying Lowpass  N=1  w0=0  Ts=Ts
      settings: SourceProductName=Control System Toolbox  SourceProductBaseCode=CT
  Gain2 : Gain  Gain=2*pi
  Product5 : Product
  Shapeit Integrator (Tustin) : Subsystem
  Shapeit Lead-Lag (Tustin) : Subsystem
  Out : Outport
  wires:
  Gain2/1 -> Discrete Varying Lowpass3/2
  Product5/1 -> Shapeit Integrator (Tustin)/1(In)
  Discrete Varying Lowpass3/1 -> Out/1
  Shapeit Integrator (Tustin)/1(Out) -> Shapeit Lead-Lag (Tustin)/1(In)
  Bus Selector/1 -> Product5/2  "<P_gain>"
  Bus Selector/2 -> Shapeit Integrator (Tustin)/2(I_fhz)  "<I_freq_hz>"
  param/1 -> Bus Selector/1
  Bus Selector/5 -> Gain2/1  "<LPF_fhz>"
  Bus Selector/4 -> Shapeit Lead-Lag (Tustin)/3(fp)  "<LL_pole_fhz>"
  reset_integrator/1 -> Shapeit Integrator (Tustin)/3(reset)
  Bus Selector/3 -> Shapeit Lead-Lag (Tustin)/2(fz)  "<LL_zero_fhz>"
  Shapeit Lead-Lag (Tustin)/1(Out) -> Discrete Varying Lowpass3/1
  In/1 -> Product5/1

== system ROPOD_Control_Control_SIM/RopodPlatformVelocityController/Platorm Velocity controller/G_I_LL_LPF Controller_theta ==
  param : Inport
  In : Inport  Port=2
  reset_integrator : Inport  Port=3
  Bus Selector : BusSelector  OutputSignals=P_gain,I_freq_hz,LL_zero_fhz,LL_pole_fhz,LPF_fhz
  Discrete Varying Lowpass3 : cstblocks/Linear Parameter Varying/Discrete Varying Lowpass  N=1  w0=0  Ts=Ts
      settings: SourceProductName=Control System Toolbox  SourceProductBaseCode=CT
  Gain2 : Gain  Gain=2*pi
  Product5 : Product
  Shapeit Integrator (Tustin) : Subsystem
  Shapeit Lead-Lag (Tustin) : Subsystem
  Out : Outport
  wires:
  Gain2/1 -> Discrete Varying Lowpass3/2
  Product5/1 -> Shapeit Integrator (Tustin)/1(In)
  Discrete Varying Lowpass3/1 -> Out/1
  Shapeit Integrator (Tustin)/1(Out) -> Shapeit Lead-Lag (Tustin)/1(In)
  Bus Selector/1 -> Product5/2  "<P_gain>"
  Bus Selector/2 -> Shapeit Integrator (Tustin)/2(I_fhz)  "<I_freq_hz>"
  param/1 -> Bus Selector/1
  Bus Selector/5 -> Gain2/1  "<LPF_fhz>"
  Bus Selector/4 -> Shapeit Lead-Lag (Tustin)/3(fp)  "<LL_pole_fhz>"
  reset_integrator/1 -> Shapeit Integrator (Tustin)/3(reset)
  Bus Selector/3 -> Shapeit Lead-Lag (Tustin)/2(fz)  "<LL_zero_fhz>"
  Shapeit Lead-Lag (Tustin)/1(Out) -> Discrete Varying Lowpass3/1
  In/1 -> Product5/1

== system ROPOD_Control_Control_SIM/RopodTorqueDistribution/ROPOD 4SW/Initialization switch ==
  ropod_cntr_mode : Inport
  curr_setp : Inport  Port=2
  Constant1 : Constant  Value=SW_COM1_MODE_TORQUE
  Constant13 : Constant  Value=SW_COM1_MODE_TORQUE
  Constant5 : Constant  Value=SW_COM1_MODE_VELOCITY
  Index Vector : MultiPortSwitch  DataPortOrder=Zero-based contiguous  zeroidx=on
  Index Vector1 : MultiPortSwitch  DataPortOrder=Zero-based contiguous  zeroidx=on
  Movinf around SW axis center : Constant  Value=[2 -2 2 -2 2 -2 2 -2]
  zeros : Constant  Value=[0 0 0 0 0 0 0 0]
  SW_cntr_mode : Outport
  wheel_setp : Outport  Port=2
  wires:
  ropod_cntr_mode/1 -> Index Vector1/1, Index Vector/1
  Constant1/1 -> Index Vector/2
  zeros/1 -> Index Vector1/2
  Index Vector1/1 -> wheel_setp/1
  Index Vector/1 -> SW_cntr_mode/1
  Constant5/1 -> Index Vector/4
  Constant13/1 -> Index Vector/3
  Movinf around SW axis center/1 -> Index Vector1/4
  curr_setp/1 -> Index Vector1/3

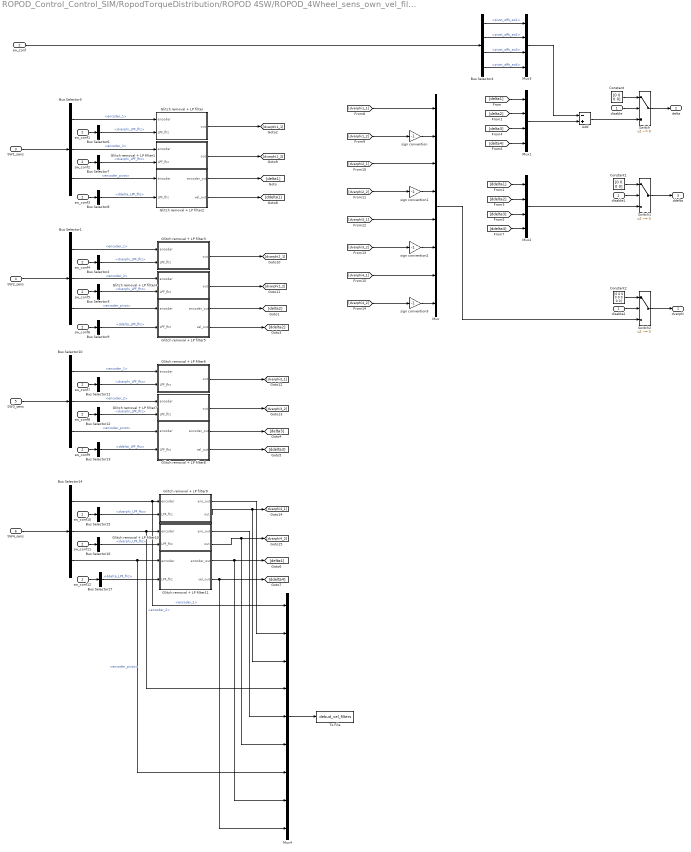
== system ROPOD_Control_Control_SIM/RopodTorqueDistribution/ROPOD 4SW/ROPOD_4Wheel_sens_own_vel_filter ==
  disable : Inport
  sw_conf : Inport  Port=2
  SW1_sens : Inport  Port=3
  SW2_sens : Inport  Port=4
  SW3_sens : Inport  Port=5
  SW4_sens : Inport  Port=6
  Add : Sum  Inputs=-+
  Bus Selector{1,5,10,14} (4 alike) : BusSelector  OutputSignals=encoder_1,encoder_2,encoder_pivot
  Bus Selector{2..3,6..7,11..12,15..16} (8 alike) : BusSelector  OutputSignals=dvarphi_LPF_fhz
  Bus Selector{8..9,13,17} (4 alike) : BusSelector  OutputSignals=ddelta_LPF_fhz
  Bus Selector4 : BusSelector  OutputSignals=pivot_offs_sw1,pivot_offs_sw2,pivot_offs_sw3,pivot_offs_sw4
  Constant : Constant  Value=[0 0 0 0]
  Constant1 : Constant  Value=[0 0 0 0]
  Constant2 : Constant  Value=[0 0 0 0 0 0 0 0]
  Glitch removal + LP filter : Subsystem
  Glitch removal + LP filter1 : Subsystem
  Glitch removal + LP filter10 : Subsystem
  Glitch removal + LP filter11 : Subsystem
  Glitch removal + LP filter2 : Subsystem
  Glitch removal + LP filter3 : Subsystem
  Glitch removal + LP filter4 : Subsystem
  Glitch removal + LP filter5 : Subsystem
  Glitch removal + LP filter6 : Subsystem
  Glitch removal + LP filter7 : Subsystem
  Glitch removal + LP filter8 : Subsystem
  Glitch removal + LP filter9 : Subsystem
  Mux : Mux  Inputs=8
  Mux1 : Mux
  Mux2 : Mux
  Mux3 : Mux
  Mux4 : Mux  Inputs=9
  Switch : Switch  Criteria=u2 ~= 0
  Switch1 : Switch  Criteria=u2 ~= 0
  Switch2 : Switch  Criteria=u2 ~= 0
  To File : ToFile  Filename=debud_vel_filters  MatrixName=debud_vel_filters
  disable1 : InportShadow
  disable2 : InportShadow
  sign convention{,1..3} (4 alike) : Gain  Gain=-1
  sw_conf{1..12} (12 alike) : InportShadow  Port=2
  dvarphi : Outport
  delta : Outport  Port=2
  ddelta : Outport  Port=3
  wires:
  SW1_sens/1 -> Bus Selector5/1
  SW2_sens/1 -> Bus Selector1/1
  [delta1] -> Mux1/1
  [delta2] -> Mux1/2
  [ddelta2] -> Mux2/2
  [ddelta1] -> Mux2/1
  SW3_sens/1 -> Bus Selector10/1
  [delta3] -> Mux1/3
  [ddelta3] -> Mux2/3
  SW4_sens/1 -> Bus Selector14/1
  [delta4] -> Mux1/4
  [ddelta4] -> Mux2/4
  Mux1/1 -> Add/2
  Mux3/1 -> Add/1
  Bus Selector4/1 -> Mux3/1  "<pivot_offs_sw1>"
  Bus Selector4/2 -> Mux3/2  "<pivot_offs_sw2>"
  Bus Selector4/3 -> Mux3/3  "<pivot_offs_sw3>"
  Bus Selector4/4 -> Mux3/4  "<pivot_offs_sw4>"
  Bus Selector5/3 -> Glitch removal + LP filter2/1(encoder)  "<encoder_pivot>"
  sign convention/1 -> Mux/2
  sign convention1/1 -> Mux/4
  sign convention2/1 -> Mux/6
  sign convention3/1 -> Mux/8
  Add/1 -> Switch/3
  Switch/1 -> delta/1
  disable/1 -> Switch/2
  Constant/1 -> Switch/1
  Switch1/1 -> ddelta/1
  Mux2/1 -> Switch1/3
  Constant1/1 -> Switch1/1
  disable1/1 -> Switch1/2
  disable2/1 -> Switch2/2
  Constant2/1 -> Switch2/1
  Mux/1 -> Switch2/3
  Switch2/1 -> dvarphi/1
  sw_conf/1 -> Bus Selector4/1
  sw_conf1/1 -> Bus Selector6/1
  sw_conf2/1 -> Bus Selector7/1
  sw_conf3/1 -> Bus Selector8/1
  sw_conf6/1 -> Bus Selector9/1
  sw_conf4/1 -> Bus Selector2/1
  sw_conf5/1 -> Bus Selector3/1
  sw_conf9/1 -> Bus Selector13/1
  sw_conf7/1 -> Bus Selector11/1
  sw_conf8/1 -> Bus Selector12/1
  sw_conf12/1 -> Bus Selector17/1
  sw_conf10/1 -> Bus Selector15/1
  sw_conf11/1 -> Bus Selector16/1
  [dvarphi1_1] -> Mux/1
  [dvarphi1_2] -> sign convention/1
  [dvarphi2_1] -> Mux/3
  [dvarphi2_2] -> sign convention1/1
  [dvarphi3_1] -> Mux/5
  [dvarphi3_2] -> sign convention2/1
  [dvarphi4_1] -> Mux/7
  [dvarphi4_2] -> sign convention3/1
  Mux4/1 -> To File/1
  Bus Selector5/1 -> Glitch removal + LP filter/1(encoder)  "<encoder_1>"
  Bus Selector6/1 -> Glitch removal + LP filter/2(LPF_fhz)  "<dvarphi_LPF_fhz>"
  Glitch removal + LP filter/1(out) -> [dvarphi1_1]
  Bus Selector7/1 -> Glitch removal + LP filter1/2(LPF_fhz)  "<dvarphi_LPF_fhz>"
  Bus Selector5/2 -> Glitch removal + LP filter1/1(encoder)  "<encoder_2>"
  Bus Selector8/1 -> Glitch removal + LP filter2/2(LPF_fhz)  "<ddelta_LPF_fhz>"
  Glitch removal + LP filter1/1(out) -> [dvarphi1_2]
  Glitch removal + LP filter2/1(encoder_out) -> [delta1]
  Glitch removal + LP filter2/2(vel_out) -> [ddelta1]
  Bus Selector2/1 -> Glitch removal + LP filter3/2(LPF_fhz)  "<dvarphi_LPF_fhz>"
  Bus Selector9/1 -> Glitch removal + LP filter5/2(LPF_fhz)  "<ddelta_LPF_fhz>"
  Bus Selector3/1 -> Glitch removal + LP filter4/2(LPF_fhz)  "<dvarphi_LPF_fhz>"
  Glitch removal + LP filter5/2(vel_out) -> [ddelta2]
  Glitch removal + LP filter3/1(out) -> [dvarphi2_1]
  Glitch removal + LP filter5/1(encoder_out) -> [delta2]
  Glitch removal + LP filter4/1(out) -> [dvarphi2_2]
  Bus Selector1/1 -> Glitch removal + LP filter3/1(encoder)  "<encoder_1>"
  Bus Selector1/2 -> Glitch removal + LP filter4/1(encoder)  "<encoder_2>"
  Bus Selector1/3 -> Glitch removal + LP filter5/1(encoder)  "<encoder_pivot>"
  Bus Selector13/1 -> Glitch removal + LP filter8/2(LPF_fhz)  "<ddelta_LPF_fhz>"
  Bus Selector10/1 -> Glitch removal + LP filter6/1(encoder)  "<encoder_1>"
  Glitch removal + LP filter7/1(out) -> [dvarphi3_2]
  Glitch removal + LP filter6/1(out) -> [dvarphi3_1]
  Bus Selector12/1 -> Glitch removal + LP filter7/2(LPF_fhz)  "<dvarphi_LPF_fhz>"
  Bus Selector10/3 -> Glitch removal + LP filter8/1(encoder)  "<encoder_pivot>"
  Glitch removal + LP filter8/1(encoder_out) -> [delta3]
  Glitch removal + LP filter8/2(vel_out) -> [ddelta3]
  Bus Selector11/1 -> Glitch removal + LP filter6/2(LPF_fhz)  "<dvarphi_LPF_fhz>"
  Bus Selector10/2 -> Glitch removal + LP filter7/1(encoder)  "<encoder_2>"
  Bus Selector17/1 -> Glitch removal + LP filter11/2(LPF_fhz)  "<ddelta_LPF_fhz>"
  Bus Selector14/1 -> Mux4/1, Glitch removal + LP filter9/1(encoder)  "<encoder_1>"
  Glitch removal + LP filter10/2(out) -> Mux4/6, [dvarphi4_2]
  Glitch removal + LP filter9/2(out) -> [dvarphi4_1], Mux4/3
  Bus Selector16/1 -> Glitch removal + LP filter10/2(LPF_fhz)  "<dvarphi_LPF_fhz>"
  Bus Selector14/3 -> Mux4/7, Glitch removal + LP filter11/1(encoder)  "<encoder_pivot>"
  Glitch removal + LP filter11/1(encoder_out) -> Mux4/8, [delta4]
  Glitch removal + LP filter11/2(vel_out) -> Mux4/9, [ddelta4]
  Bus Selector15/1 -> Glitch removal + LP filter9/2(LPF_fhz)  "<dvarphi_LPF_fhz>"
  Bus Selector14/2 -> Mux4/4, Glitch removal + LP filter10/1(encoder)  "<encoder_2>"
  Glitch removal + LP filter9/1(enc_out) -> Mux4/2
  Glitch removal + LP filter10/1(enc_out) -> Mux4/5
